simulink model "model1"  (R2021b)
settings: Solver=VariableStepAuto  StartTime=0.0  StopTime=30.0  RelTol=1e-3
values from neighbouring files (symbols this model uses):
  d = 2    [a2q2.m]
undefined symbols (not defined in the file or in its folder): A, B
settings Model: SnapshotBufferSize=30  SnapshotInterval=30  Creator=Clement_Wu  LastModifiedBy=Clement_Wu

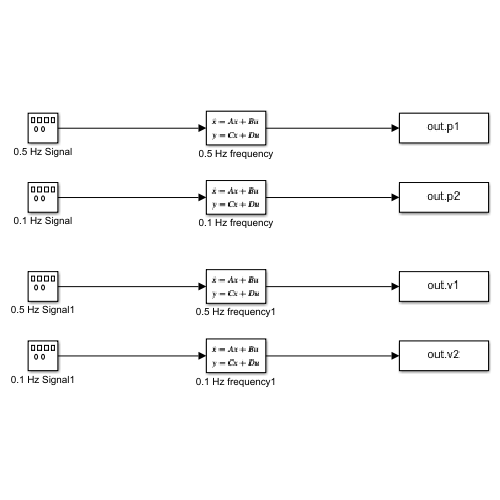
[thumbnail: Simulink's stored preview of the top-level diagram]
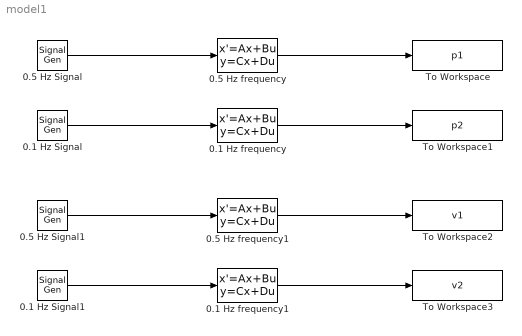
== system model1 ==
  0.1 Hz Signal : SignalGenerator  WaveForm=square  Frequency=0.1
  0.1 Hz Signal1 : SignalGenerator  WaveForm=square  Frequency=0.1
  0.1 Hz frequency : StateSpace  A=A  B=B  C=[1 0]  D=d  InitialCondition=0  ContinuousStateAttributes='x'
  0.1 Hz frequency1 : StateSpace  A=A  B=B  C=[0 1]  D=d  InitialCondition=0  ContinuousStateAttributes='x'
  0.5 Hz Signal : SignalGenerator  WaveForm=square  Frequency=0.5
  0.5 Hz Signal1 : SignalGenerator  WaveForm=square  Frequency=0.5
  0.5 Hz frequency : StateSpace  A=A  B=B  C=[1 0]  D=d  InitialCondition=0  ContinuousStateAttributes='x'
  0.5 Hz frequency1 : StateSpace  A=A  B=B  C=[0 1]  D=d  InitialCondition=0  ContinuousStateAttributes='x'
  To Workspace : ToWorkspace  VariableName=p1  SaveFormat=Timeseries  SampleTime=-1
  To Workspace1 : ToWorkspace  VariableName=p2  SaveFormat=Timeseries  SampleTime=-1
  To Workspace2 : ToWorkspace  VariableName=v1  SaveFormat=Timeseries  SampleTime=-1
  To Workspace3 : ToWorkspace  VariableName=v2  SaveFormat=Timeseries  SampleTime=-1
  wires:
  0.5 Hz frequency/1 -> To Workspace/1
  0.1 Hz Signal/1 -> 0.1 Hz frequency/1
  0.1 Hz frequency/1 -> To Workspace1/1
  0.5 Hz Signal/1 -> 0.5 Hz frequency/1
  0.5 Hz Signal1/1 -> 0.5 Hz frequency1/1
  0.1 Hz Signal1/1 -> 0.1 Hz frequency1/1
  0.1 Hz frequency1/1 -> To Workspace3/1
  0.5 Hz frequency1/1 -> To Workspace2/1
